simulink model "POINTING_1"  (R2025b)
settings: Solver=ode45  StartTime=0.0  StopTime=20  RelTol=1e-3
values from neighbouring files (symbols this model uses):
  J = 0.002    [Reaction_Wheel_sim.m]    (also in SIMULINK_InitialParameters.m; compare_PD_LQR.m = 0.000634)
  Jw = 1e-5    (= 1e-05)    [Reaction_Wheel_sim.m]    (also in SIMULINK_InitialParameters.m; compare_PD_LQR.m = 4.607e-05)
  Kd = 0.02    [Reaction_Wheel_sim.m]    (also in SIMULINK_InitialParameters.m = 0.01)
  Kp = 0.05    [Reaction_Wheel_sim.m]    (also in SIMULINK_InitialParameters.m = 0.02)
  omega0 = deg2rad( 20 * (2*rand-1) )    [Reaction_Wheel_sim.m]    (also in SIMULINK_InitialParameters.m = deg2rad(8); compare_PD_LQR.m = deg2rad(8))
  theta0 = deg2rad( rand*360 - 180 )    [Reaction_Wheel_sim.m]    (also in SIMULINK_InitialParameters.m = deg2rad(15); compare_PD_LQR.m = deg2rad(15))
  theta_ref = deg2rad(theta_ref_deg)    [Reaction_Wheel_sim.m]    (also in SIMULINK_InitialParameters.m; compare_PD_LQR.m)
settings Model: Creator=bbtp  LastModifiedBy=bbtp

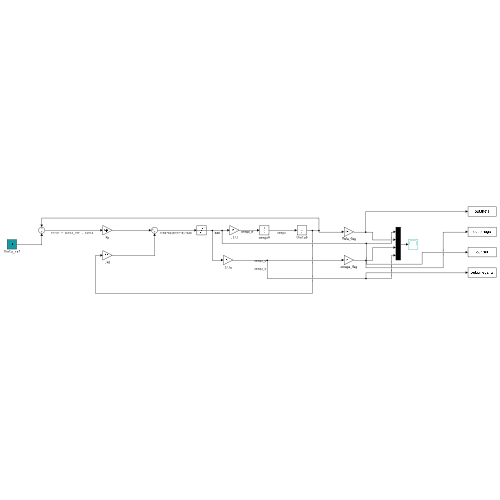
[thumbnail: Simulink's stored preview of the top-level diagram]
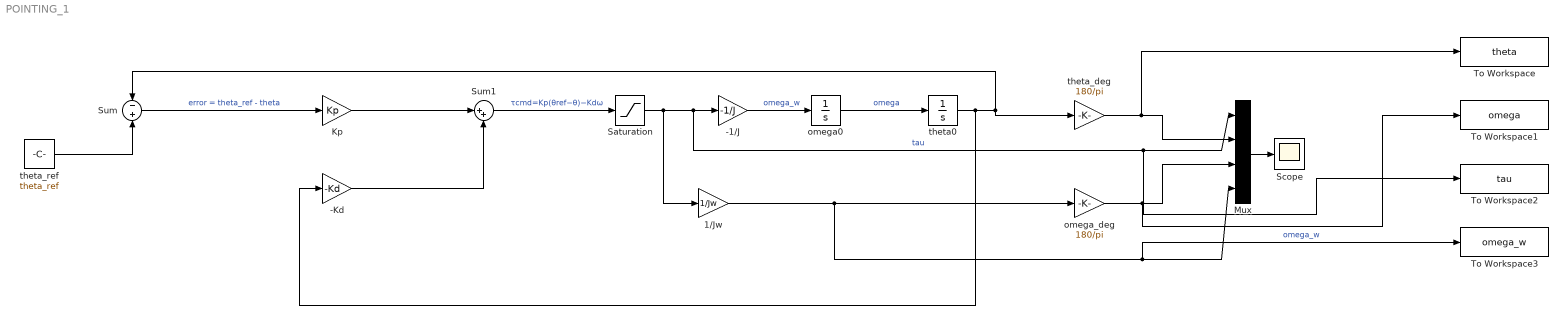
== system POINTING_1 ==
  -1/J : Gain  Gain=-1/J
  -Kd : Gain  Gain=-Kd
  1/Jw : Gain  Gain=1/Jw
  Kp : Gain  Gain=Kp
  Mux : Mux
  Saturation : Saturate
  Scope : Scope
      settings: ActiveDisplayYMinimum=-411567.73029706057  ActiveDisplayYMaximum=343540.60888628056
  Sum : Sum  Inputs=-+
  Sum1 : Sum  Inputs=|++
  To Workspace : ToWorkspace  VariableName=theta  SaveFormat=Timeseries  SampleTime=-1
  To Workspace1 : ToWorkspace  VariableName=omega  SaveFormat=Timeseries  SampleTime=-1
  To Workspace2 : ToWorkspace  VariableName=tau  SaveFormat=Timeseries  SampleTime=-1
  To Workspace3 : ToWorkspace  VariableName=omega_w  SaveFormat=Timeseries  SampleTime=-1
  omega0 : Integrator  InitialCondition=omega0
  omega_deg : Gain  Gain=180/pi
  theta0 : Integrator  InitialCondition=theta0
  theta_deg : Gain  Gain=180/pi
  theta_ref : Constant  Value=theta_ref
  wires:
  Sum/1 -> Kp/1  "error = theta_ref - theta"
  Kp/1 -> Sum1/1
  -Kd/1 -> Sum1/2
  Sum1/1 -> Saturation/1  "τcmd​=Kp​(θref​−θ)−Kd​ω"
  Saturation/1 -> 1/Jw/1, To Workspace2/1, Mux/1, -1/J/1  "tau"
  omega0/1 -> theta0/1  "omega"
  theta_ref/1 -> Sum/2
  1/Jw/1 -> To Workspace3/1, Mux/4, omega_deg/1  "omega_w"
  Mux/1 -> Scope/1
  theta_deg/1 -> To Workspace/1, Mux/2
  omega_deg/1 -> To Workspace1/1, Mux/3
  -1/J/1 -> omega0/1  "omega_w"
  theta0/1 -> -Kd/1, Sum/1, theta_deg/1
